simulink model "sldemo_mdlref_counter_bus"  (Simulink 7.6)
settings: Solver=FixedStepDiscrete  StartTime=0.0  StopTime=30.0  FixedStep=0.1  RelTol=1e-3
PreLoadFcn:
  | load sldemo_mdlref_counter_bus.mat
settings Model: Creator=The MathWorks Inc.  ExtModeAutoUpdateStatusClock=off
settings DataIOCC: ExternalInput=topOut.COUNTERBUS  LoadExternalInput=on  SaveFormat=StructureWithTime  SaveOutput=off  SaveTime=off  SignalLoggingName=subOut
settings OptimizationCC: InlineParams=on  InlineInvariantSignals=on  InitFltsAndDblsToZero=on  BufferReusableBoundary=off
settings DebuggingCC: SaveWithParameterizedLinksMsg=none  CheckExecutionContextPreStartOutputMsg=on  CheckExecutionContextRuntimeOutputMsg=on  SolverPrmCheckMsg=none  MultiTaskDSMMsg=warning  MultiTaskCondExecSysMsg=none  SigSpecEnsureSampleTimeMsg=none  BusObjectLabelMismatch=error  ModelReferenceDataLoggingMessage=none  StrictBusMsg=ErrorOnBusTreatedAsVector
settings HardwareCC: TargetHWDeviceType=32-bit Generic
settings ModelReferenceCC: UpdateModelReferenceTargets=IfOutOfDate  CheckModelReferenceTargetMessage=none
settings RTWCC: GenerateReport=on  ProcessScript=grt_make_rtw_hook  LaunchReport=on  IncludeERTFirstTime=on
settings CodeAppCC: MaxIdLength=100
settings GRTTargetCC: TargetFcnLib=ansi_tfl_tmw.mat

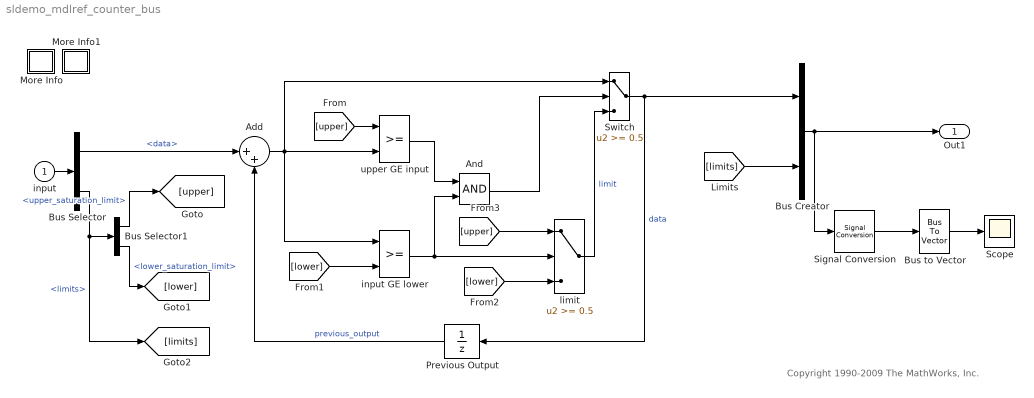
== system sldemo_mdlref_counter_bus ==
  note: Copyright 1990-2009 The MathWorks, Inc.
  " input" : Inport  OutDataTypeStr=Bus: COUNTERBUS  BusOutputAsStruct=on
  " input GE lower" : RelationalOperator  Priority=1  InputSameDT=on
      settings: AttributesFormatString=\n
  " limit" : Switch  Threshold=0.5  SaturateOnIntegerOverflow=on  InputSameDT=on
  Add : Sum  Inputs=|++
  And : Logic
  Bus Creator : BusCreator  Inputs=2  OutDataTypeStr=Bus: COUNTERBUS  NonVirtualBus=on
  Bus Selector : BusSelector  OutputSignals=data,limits
  Bus Selector1 : BusSelector  OutputSignals=upper_saturation_limit,lower_saturation_limit
  Bus to Vector : BusToVector
  More Info : Subsystem
      settings: OpenFcn=showdemo('sldemo_mdlref_bus')
      mask Display: disp('?')
  More Info1 : Subsystem
      settings: OpenFcn=|
      | html = fullfile(matlabroot, 'toolbox', 'simulink', 'simdemos', 'simfeatures', 'html', 'sldemo_mdlref_protect.html');
      | 
      | if(isempty(dir(html)))                                                                      error('simdemos:sldemo_mdlref_counter_bus:notFound','"%s" not found.',html);
      | else
      |    web(html, '-helpbrowser');
      | end
      mask Display: disp('?')
  Previous Output : UnitDelay  SampleTime=-1
  Scope : Scope
      settings: TimeRange=30  YMin=0  YMax=40
  Signal Conversion : SignalConversion  ConversionOutput=Virtual bus
  Switch : Switch  Threshold=0.5  SaturateOnIntegerOverflow=on  InputSameDT=on
  upper GE input : RelationalOperator  Priority=0  InputSameDT=on
      settings: AttributesFormatString=\n
  Out1 : Outport  OutDataTypeStr=Bus: COUNTERBUS
  wires:
  [upper] -> " limit"/1
  Switch/1 -> Previous Output/1, Bus Creator/1  "data"
  " limit"/1 -> Switch/3  "limit"
  upper GE input/1 -> And/1
  Previous Output/1 -> Add/2  "previous_output"
  [lower] -> " limit"/3
  [upper] -> upper GE input/1
  [lower] -> " input GE lower"/2
  " input GE lower"/1 -> And/2, " limit"/2
  And/1 -> Switch/2
  Add/1 -> " input GE lower"/1, upper GE input/2, Switch/1
  " input"/1 -> Bus Selector/1
  Bus Selector/2 -> Bus Selector1/1, [limits]  "<limits>"
  Bus Selector/1 -> Add/1  "<data>"
  Bus Selector1/1 -> [upper]  "<upper_saturation_limit>"
  Bus Selector1/2 -> [lower]  "<lower_saturation_limit>"
  Bus Creator/1 -> Out1/1, Signal Conversion/1
  [limits] -> Bus Creator/2
  Signal Conversion/1 -> Bus to Vector/1
  Bus to Vector/1 -> Scope/1

== system sldemo_mdlref_counter_bus/More Info ==

== system sldemo_mdlref_counter_bus/More Info1 ==
